simulink model "test_onoff_button"  (R2022b)
settings: Solver=FixedStepAuto  StartTime=0.0  StopTime=240  FixedStep=0.1  RelTol=1e-3
settings Model: Creator=alewi  LastModifiedBy=cristian
settings ConfigComp: CovEnable=on  RecordCoverage=on  CovModelRefEnable=on

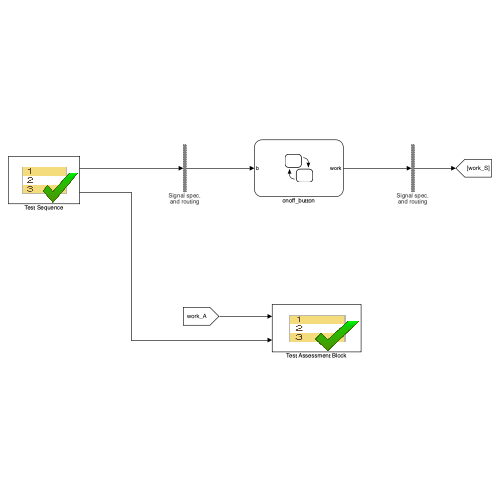
[thumbnail: Simulink's stored preview of the top-level diagram]
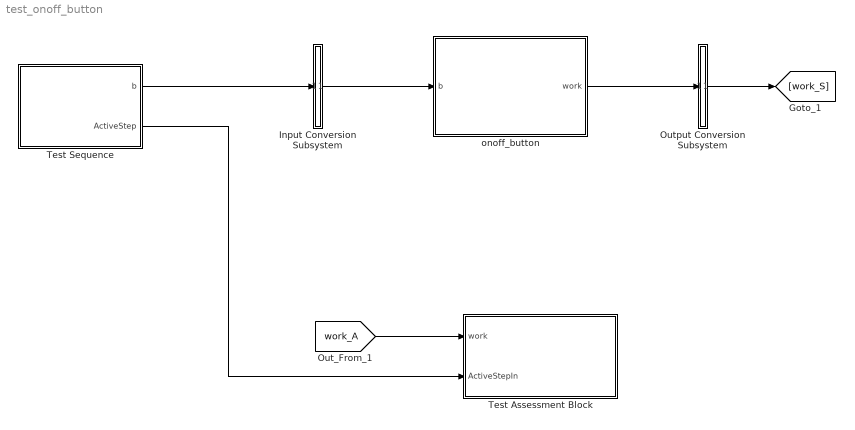
== system test_onoff_button ==
  Input Conversion Subsystem : Subsystem  Tag=__SLT_ICS__  Description=|
      | Signal spec.
      | and routing
      settings: AttributesFormatString=%<Description>
  Output Conversion Subsystem : Subsystem  Tag=__SLT_OCS__  Description=|
      | Signal spec.
      | and routing
      settings: AttributesFormatString=%<Description>
  Test Assessment Block : Test Sequence  Tag=__SLT_ASMT__  TreatAsAtomicUnit=on
  Test Sequence : Test Sequence  TreatAsAtomicUnit=on
  onoff_button : Stateflow chart  TreatAsAtomicUnit=on
  wires:
  Output Conversion Subsystem/1(Outport_1) -> [work_S]
  Input Conversion Subsystem/1(Outport_1) -> onoff_button/1(b)
  onoff_button/1(work) -> Output Conversion Subsystem/1(Inport_1)
  Test Sequence/1(b) -> Input Conversion Subsystem/1(Inport_1)
  Test Sequence/2(ActiveStep) -> Test Assessment Block/2(ActiveStepIn)
  [work_A] -> Test Assessment Block/1(work)

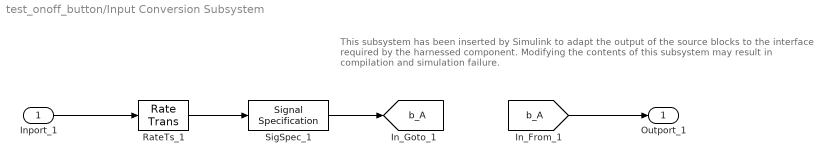
== system test_onoff_button/Input Conversion Subsystem ==
  note: This subsystem has been inserted by Simulink to adapt the output of the source blocks to the interface required by the harnessed component.
      |  Modifying the contents of this subsystem may result in compilation and simulation failure.
  Inport_1 : Inport
  RateTs_1 : RateTransition  OutPortSampleTime=[-1, 0]
  SigSpec_1 : SignalSpecification  OutDataTypeStr=boolean  Dimensions=[1]  SampleTime=[-1, 0]
  Outport_1 : Outport
  tag scope: b_A=global
  wires:
  [b_A] -> Outport_1/1
  SigSpec_1/1 -> [b_A]
  RateTs_1/1 -> SigSpec_1/1
  Inport_1/1 -> RateTs_1/1

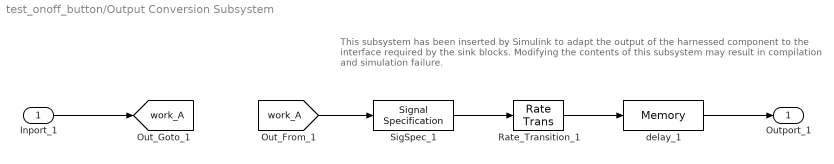
== system test_onoff_button/Output Conversion Subsystem ==
  note: This subsystem has been inserted by Simulink to adapt the output of the harnessed component to the interface required by the sink blocks.
      |  Modifying the contents of this subsystem may result in compilation and simulation failure.
  Inport_1 : Inport
  Rate_Transition_1 : RateTransition  OutPortSampleTimeOpt=Inherit
  SigSpec_1 : SignalSpecification  OutDataTypeStr=boolean  Dimensions=[1]
  delay_1 : Memory
  Outport_1 : Outport
  tag scope: work_A=global
  wires:
  Inport_1/1 -> [work_A]
  [work_A] -> SigSpec_1/1
  SigSpec_1/1 -> Rate_Transition_1/1
  Rate_Transition_1/1 -> delay_1/1
  delay_1/1 -> Outport_1/1

== stateflow chart test_onoff_button/Test Assessment Block ==
  state LegitBehavior
    state Run
      state Verify_LB_Init
        verify(work == 0);
      state Verify_LB_Press
        verify(work == 1);
      state Verify_CB_Release
        verify(work == 1);
      state Verify_LB_LongPress
        verify(work == 1);
      state Verify_LB_ReleaseLongPression
        verify(work == 0);
      state Verify_LB_Void
      (junction 388) -> (junction 391) [order 2]
      (junction 387) -> (junction 388) [order 1] : [ActiveStepIn == ActiveStepEnumH2.LB_Init
          | ]
      (junction 388) -> Verify_LB_Init [order 1] : [~in(LegitBehavior.Run.Verify_LB_Init)]
      (junction 94) -> Verify_LB_Press [order 1] : [~in(LegitBehavior.Run.Verify_LB_Press)]
      (junction 84) -> (junction 94) [order 1] : [ActiveStepIn == ActiveStepEnumH2.LB_Press
          | ]
      (junction 94) -> (junction 97) [order 2]
      (junction 84) -> (junction 101) [order 2]
      (junction 101) -> (junction 102) [order 1] : [ActiveStepIn == ActiveStepEnumH2.LB_Release
          | ]
      (junction 102) -> Verify_CB_Release [order 1] : [~in(LegitBehavior.Run.Verify_CB_Release)]
      (junction 101) -> (junction 356) [order 2]
      (junction 102) -> (junction 105) [order 2]
      (junction 356) -> (junction 357) [order 1] : [ActiveStepIn == ActiveStepEnumH2.LB_LongPress
          | ]
      (junction 357) -> Verify_LB_LongPress [order 1] : [~in(LegitBehavior.Run.Verify_LB_LongPress)]
      (junction 356) -> (junction 139) [order 2]
      (junction 357) -> (junction 360) [order 2]
      (junction 139) -> (junction 140) [order 1] : [ActiveStepIn == ActiveStepEnumH2.LB_ReleaseLongPression
          | ]
      (junction 140) -> Verify_LB_ReleaseLongPression [order 1] : [~in(LegitBehavior.Run.Verify_LB_ReleaseLongPression)]
      (junction 139) -> (junction 148) [order 2]
      (junction 140) -> (junction 143) [order 2]
      (junction 148) -> (junction 149)
      (junction 149) -> LegitBehavior.Run.Verify_LB_Void [order 1] : [~in(LegitBehavior.Run.Verify_LB_Void)]
      (junction 149) -> (junction 152) [order 2]
      (junction 387) -> (junction 84) [order 2]
      LegitBehavior.Run -> (junction 387)
      (default) -> (junction 387)
    (default) -> LegitBehavior.Run
  state CompleteBehavior
    state Run
      state Verify_CB_Init
        verify(work == 0);
      state Verify_CB_Inactive_Wait
        verify(work == 0);
      state Verify_CB_Inactive_Pressed
        verify(work == 1);
      state Verify_CB_Active_Wait
        verify(work == 1);
      state Verify_CB_Active_Pressed
        verify(work == 1);
      state Verify_CB_Active_Released
        verify(work == 1);
      state Verify_CB_Active_PressedAgain
        verify(work == 1);
      state Verify_CB_Active_LongPressed
        verify(work == 1);
      state Verify_CB_Active_NoWork
        verify(work == 0);
      state Verify_CB_Backto_Inactive
        verify(work == 0);
      state Verify_CB_Void
      (default) -> (junction 180)
      CompleteBehavior.Run -> (junction 180)
      (junction 180) -> (junction 181) [order 1] : [ActiveStepIn == ActiveStepEnumH2.CB_Init
          | ]
      (junction 181) -> Verify_CB_Init [order 1] : [~in(CompleteBehavior.Run.Verify_CB_Init)]
      (junction 180) -> (junction 189) [order 2]
      (junction 181) -> (junction 184) [order 2]
      (junction 189) -> (junction 190) [order 1] : [ActiveStepIn == ActiveStepEnumH2.CB_Inactive_Wait
          | ]
      (junction 190) -> Verify_CB_Inactive_Wait [order 1] : [~in(CompleteBehavior.Run.Verify_CB_Inactive_Wait)]
      (junction 189) -> (junction 252) [order 2]
      (junction 190) -> (junction 193) [order 2]
      (junction 252) -> (junction 253) [order 1] : [ActiveStepIn == ActiveStepEnumH2.CB_Inactive_Pressed
          | ]
      (junction 253) -> Verify_CB_Inactive_Pressed [order 1] : [~in(CompleteBehavior.Run.Verify_CB_Inactive_Pressed)]
      (junction 252) -> (junction 270) [order 2]
      (junction 253) -> (junction 256) [order 2]
      (junction 270) -> (junction 271) [order 1] : [ActiveStepIn == ActiveStepEnumH2.CB_Active_Wait
          | ]
      (junction 271) -> Verify_CB_Active_Wait [order 1] : [~in(CompleteBehavior.Run.Verify_CB_Active_Wait)]
      (junction 270) -> (junction 288) [order 2]
      (junction 271) -> (junction 274) [order 2]
      (junction 288) -> (junction 289) [order 1] : [ActiveStepIn == ActiveStepEnumH2.CB_Active_Pressed
          | ]
      (junction 289) -> Verify_CB_Active_Pressed [order 1] : [~in(CompleteBehavior.Run.Verify_CB_Active_Pressed)]
      (junction 288) -> (junction 297) [order 2]
      (junction 289) -> (junction 292) [order 2]
      (junction 297) -> (junction 298) [order 1] : [ActiveStepIn == ActiveStepEnumH2.CB_Active_Released
          | ]
      (junction 298) -> Verify_CB_Active_Released [order 1] : [~in(CompleteBehavior.Run.Verify_CB_Active_Released)]
      (junction 297) -> (junction 306) [order 2]
      (junction 298) -> (junction 301) [order 2]
      (junction 306) -> (junction 307) [order 1] : [ActiveStepIn == ActiveStepEnumH2.CB_Active_PressedAgain
          | ]
      (junction 307) -> Verify_CB_Active_PressedAgain [order 1] : [~in(CompleteBehavior.Run.Verify_CB_Active_PressedAgain)]
      (junction 306) -> (junction 315) [order 2]
      (junction 307) -> (junction 310) [order 2]
      (junction 315) -> (junction 316) [order 1] : [ActiveStepIn == ActiveStepEnumH2.CB_Active_LongPressed
          | ]
      (junction 316) -> Verify_CB_Active_LongPressed [order 1] : [~in(CompleteBehavior.Run.Verify_CB_Active_LongPressed)]
      (junction 345) -> (junction 333) [order 2]
      (junction 316) -> (junction 319) [order 2]
      (junction 345) -> (junction 346) [order 1] : [ActiveStepIn == ActiveStepEnumH2.CB_Active_NoWork
          | ]
      (junction 346) -> Verify_CB_Active_NoWork [order 1] : [~in(CompleteBehavior.Run.Verify_CB_Active_NoWork)]
      (junction 333) -> (junction 334) [order 1] : [ActiveStepIn == ActiveStepEnumH2.CB_Backto_Inactive
          | ]
      (junction 334) -> Verify_CB_Backto_Inactive [order 1] : [~in(CompleteBehavior.Run.Verify_CB_Backto_Inactive)]
      (junction 333) -> (junction 260) [order 2]
      (junction 334) -> (junction 337) [order 2]
      (junction 260) -> (junction 261)
      (junction 261) -> Verify_CB_Void [order 1] : [~in(CompleteBehavior.Run.Verify_CB_Void)]
      (junction 261) -> (junction 264) [order 2]
      (junction 346) -> (junction 349) [order 2]
      (junction 315) -> (junction 345) [order 2]
    (default) -> CompleteBehavior.Run
  state WrongPressionBehavior
    state Run
      state Verify_WB_Init
        verify(work == 0);
      state Verify_WB_Press
        verify(work == 1);
      state Verify_WB_Release
        verify(work == 1);
      state Verify_WB_LongPress
        verify(work == 1);
      state Verify_WB_Backto_Wait
        verify(work == 1);
      state Verify_LB_Void
      (default) -> (junction 404)
      WrongPressionBehavior.Run -> (junction 404)
      (junction 404) -> (junction 405) [order 1] : [ActiveStepIn == ActiveStepEnumH2.WB_Init
          | ]
      (junction 405) -> Verify_WB_Init [order 1] : [~in(WrongPressionBehavior.Run.Verify_WB_Init)]
      (junction 404) -> (junction 413) [order 2]
      (junction 405) -> (junction 408) [order 2]
      (junction 413) -> (junction 414) [order 1] : [ActiveStepIn == ActiveStepEnumH2.WB_Press
          | ]
      (junction 414) -> Verify_WB_Press [order 1] : [~in(WrongPressionBehavior.Run.Verify_WB_Press)]
      (junction 413) -> (junction 421) [order 2]
      (junction 414) -> (junction 417) [order 2]
      (junction 421) -> (junction 422) [order 1] : [ActiveStepIn == ActiveStepEnumH2.WB_Release
          | ]
      (junction 422) -> Verify_WB_Release [order 1] : [~in(WrongPressionBehavior.Run.Verify_WB_Release)]
      (junction 421) -> (junction 429) [order 2]
      (junction 422) -> (junction 425) [order 2]
      (junction 429) -> (junction 430) [order 1] : [ActiveStepIn == ActiveStepEnumH2.WB_LongPress
          | ]
      (junction 430) -> Verify_WB_LongPress [order 1] : [~in(WrongPressionBehavior.Run.Verify_WB_LongPress)]
      (junction 429) -> (junction 437) [order 2]
      (junction 430) -> (junction 433) [order 2]
      (junction 437) -> (junction 438) [order 1] : [ActiveStepIn == ActiveStepEnumH2.WB_Backto_Wait
          | ]
      (junction 438) -> Verify_WB_Backto_Wait [order 1] : [~in(WrongPressionBehavior.Run.Verify_WB_Backto_Wait)]
      (junction 438) -> (junction 441) [order 2]
      (junction 446) -> (junction 447)
      (junction 447) -> WrongPressionBehavior.Run.Verify_LB_Void [order 1] : [~in(WrongPressionBehavior.Run.Verify_LB_Void)]
      (junction 447) -> (junction 450) [order 2]
      (junction 437) -> (junction 446) [order 2]
    (default) -> WrongPressionBehavior.Run
  (default) -> LegitBehavior [order 1] : [Active_Scenario_Index == 1]
  (default) -> CompleteBehavior [order 2] : [Active_Scenario_Index == 2]
  (default) -> WrongPressionBehavior [order 3] : {assert(Active_Scenario_Index == 3,'The value of Scenario Parameter ''Active_Scenario_Index'' is not valid. Use the index of the scenario to specify it.')}
  data: work input boolean size=[1]; ActiveStepIn input; Active_Scenario_Index parameter =2

== stateflow chart test_onoff_button/onoff_button ==
  note: Stato di accensione del bottone onoff
  note: In questo stato il bottone può accendere la macchina
  state INACTIVE
    state Pressed
      en: work = HIGH
    state Wait
      en: work = LOW
    (default) -> INACTIVE.Wait
    INACTIVE.Wait -> INACTIVE.Pressed : [b == PRESSED]
  note: Stato di spegnimento del bottone onoff
  note: In questo stato il bottone può spengere la macchina
  state ACTIVE
    state Wait
      en:
      b_long = RELEASED
    state Pressed
      en:
      b_long = RELEASED;
      on after(DURATION,sec): b_long = PRESSED
    state LongPressed
      en: work = LOW;
    (default) -> ACTIVE.Wait
    ACTIVE.Wait -> ACTIVE.Pressed : [b == PRESSED]
    ACTIVE.Pressed -> ACTIVE.Wait [order 1] : [b == RELEASED]
    ACTIVE.Pressed -> LongPressed [order 2] : [b_long == PRESSED && b == PRESSED]
  note: Se il bottone viene premuto una sola volta, il sistema viene acceso.
      | Se il bottone viene premuto per 1 secondo, il sistema viene spento.
      | Una pressione prolungata senza rilascio del bottone, non causa un alternarsi di accensioni e spegnimenti continui.
  (default) -> INACTIVE
  INACTIVE.Pressed -> ACTIVE : [b == RELEASED]
  LongPressed -> INACTIVE : [b==RELEASED]
  data: PRESSED constant boolean size=1 =0; RELEASED constant boolean size=1 =1; b input boolean size=1; DURATION constant double size=1 =1; b_long local boolean size=1; HIGH constant boolean size=1 =1; LOW constant boolean size=1 =0; work output boolean size=1

== stateflow chart test_onoff_button/Test Sequence ==
  settings: updateMethod=DISCRETE  sampleTime=0.1
  state LegitBehavior
    state LB_Init
      b = true
    state LB_Press
      b = false
      settings: description=|
          | Il bottone viene premuto per la prima volta.
          | L'output in questo caso è alto alla singola pressione.
          | Indipendentemente dal tempo in cui permango, non dovrei cambiare stato.
    state LB_Release
      b = true
      settings: description=|
          | Il bottone viene rilasciato.
          | Il sistema dovrebbe prepararsi al comportamento di un bottone a livelli, quindi cambia stato.
    state LB_LongPress
      b = false
      settings: description=|
          | Pressione prolungata, dopo DURATION secondi (1, in questo caso) dovrei ottenere l'output in uscita.
          | Mi mantengo in pressione per il tempo necessario all'impostazione dell'output, più un sample time.
    state LB_ReleaseLongPression
      b = false
      settings: description=|
          | Rilascio il bottone dopo la pressione prolungata.
          | Il sistema dovrebbe preparasi al comportamento di un bottone semplice.
    state LB_Backto_Inactive
      b = true
    (default) -> LB_Init
    LB_Init -> LB_Press : [
        | true
        | ]
    LB_Press -> LB_Release : [
        | after(sample_time, sec)
        | ]
    LB_Release -> LB_LongPress : [
        | true
        | ]
    LB_LongPress -> LB_ReleaseLongPression : [
        | after(1+sample_time, sec)
        | ]
    LB_ReleaseLongPression -> LB_Backto_Inactive : [
        | true
        | ]
  state CompleteBehavior
    state CB_Init
      b = true
      settings: description=Stato iniziale, nessuna pressione effettuata.\
    state CB_Inactive_Wait
      b = true
    state CB_Inactive_Pressed
      b = false
      settings: description=Il bottone viene premuto, mi apetto alto il segnale di work.
    state CB_Active_Wait
      b = true
      settings: description=Rilascio e permango in fase di attesa per lo spegnimento.
    state CB_Active_Pressed
      b = false
      settings: description=Effettuo la pressione per un singolo istante di campionamento.
    state CB_Active_Released
      b = true
      settings: description=Pressione troppo corta, ritorno nello stato precedente
    state CB_Active_PressedAgain
      b  = false.
      settings: description=Avvio una nuova pressione.
    state CB_Active_LongPressed
      b = false
      settings: description=Pressione prolungata al fine di effettuare lo spegnimento.
    state CB_Active_NoWork
      b = false
      settings: description=Rilascio il bottone per ritornare in attesa di accensione
    state CB_Backto_Inactive
      b = true
    (default) -> CB_Init
    CB_Init -> CB_Inactive_Wait : [
        | true
        | ]
    CB_Inactive_Wait -> CB_Inactive_Pressed : [
        | true
        | ]
    CB_Inactive_Pressed -> CB_Active_Wait : [
        | true
        | ]
    CB_Active_Wait -> CB_Active_Pressed : [
        | true
        | ]
    CB_Active_Pressed -> CB_Active_Released : [
        | true
        | ]
    CB_Active_Released -> CB_Active_PressedAgain : [
        | true
        | ]
    CB_Active_PressedAgain -> CB_Active_LongPressed : [
        | true
        | ]
    CB_Active_LongPressed -> CB_Active_NoWork : [
        | after(1,sec)
        | ]
    CB_Active_NoWork -> CB_Backto_Inactive : [
        | true
        | ]
  state WrongPressionBehavior
    state WB_Init
      b = true
    state WB_Press
      b = false
      settings: description=|
          | Il bottone viene premuto per la prima volta.
          | L'output in questo caso è alto alla singola pressione.
          | Indipendentemente dal tempo in cui permango, non dovrei cambiare stato.
    state WB_Release
      b = true
      settings: description=|
          | Il bottone viene rilasciato.
          | Il sistema dovrebbe prepararsi al comportamento di un bottone a livelli, quindi cambia stato.
    state WB_LongPress
      b = false
      settings: description=Pressione prolungata ma troppo corta.
    state WB_Backto_Wait
      b = true
    (default) -> WB_Init
    WB_Init -> WB_Press : [
        | true
        | ]
    WB_Press -> WB_Release : [
        | after(sample_time, sec)
        | ]
    WB_Release -> WB_LongPress : [
        | true
        | ]
    WB_LongPress -> WB_Backto_Wait : [
        | after(0.5, sec)
        | ]
  (default) -> LegitBehavior [order 1] : [Active_Scenario_Index == 1]
  (default) -> CompleteBehavior [order 2] : [Active_Scenario_Index == 2]
  (default) -> WrongPressionBehavior [order 3] : {assert(Active_Scenario_Index == 3,'The value of Scenario Parameter ''Active_Scenario_Index'' is not valid. Use the index of the scenario to specify it.')}
  data: b output boolean size=[1]; Active_Scenario_Index parameter =2; ActiveStep output Enum: ActiveStepEnumH2; sample_time constant double =str2num(get_param('InductionCooker','FixedStep'))
